simulink model "syt_a23"  (Simulink 7.0)
settings: Solver=ode3  StartTime=0.0  StopTime=10.0  FixedStep=0.01  RelTol=1e-3
settings Model: Creator=LAT04  LastModifiedBy=LAT04

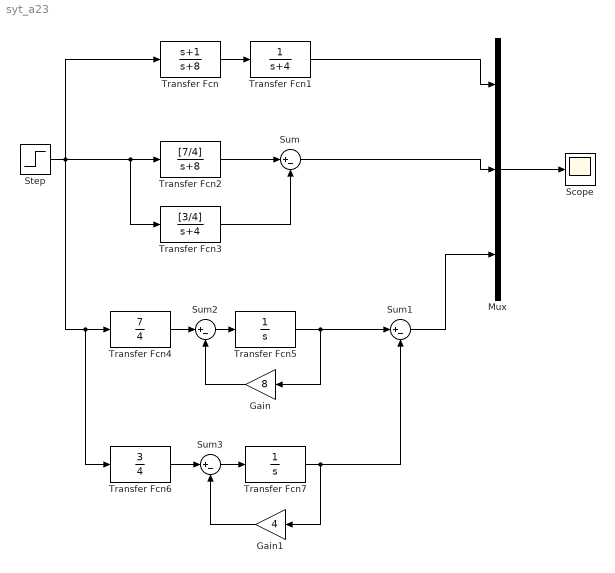
== system syt_a23 ==
  Gain : Gain  Orientation=left  Gain=8  ParameterDataType=sfix(16)  ParameterScaling=2^0  OutDataType=sfix(16)  OutScaling=2^0
  Gain1 : Gain  Orientation=left  Gain=4  ParameterDataType=sfix(16)  ParameterScaling=2^0  OutDataType=sfix(16)  OutScaling=2^0
  Mux : Mux  Inputs=3
  Scope : Scope
  Step : Step  SampleTime=0
  Sum{,1..3} (4 alike) : Sum  Inputs=|+-  OutDataType=sfix(16)  OutScaling=2^0
  Transfer Fcn : TransferFcn  Numerator=[1 1]  Denominator=[1 8]
  Transfer Fcn1 : TransferFcn  Denominator=[1 4]
  Transfer Fcn2 : TransferFcn  Numerator=[7/4]  Denominator=[1 8]
  Transfer Fcn3 : TransferFcn  Numerator=[3/4]  Denominator=[1 4]
  Transfer Fcn4 : TransferFcn  Numerator=[7]  Denominator=[4]
  Transfer Fcn5 : TransferFcn  Denominator=[1 0]
  Transfer Fcn6 : TransferFcn  Numerator=[3]  Denominator=[4]
  Transfer Fcn7 : TransferFcn  Denominator=[1 0]
  wires:
  Step/1 -> Transfer Fcn/1, Transfer Fcn2/1, Transfer Fcn3/1, Transfer Fcn4/1, Transfer Fcn6/1
  Transfer Fcn/1 -> Transfer Fcn1/1
  Transfer Fcn1/1 -> Mux/1
  Transfer Fcn2/1 -> Sum/1
  Transfer Fcn3/1 -> Sum/2
  Sum2/1 -> Transfer Fcn5/1
  Transfer Fcn4/1 -> Sum2/1
  Transfer Fcn5/1 -> Gain/1, Sum1/1
  Gain/1 -> Sum2/2
  Transfer Fcn6/1 -> Sum3/1
  Sum3/1 -> Transfer Fcn7/1
  Gain1/1 -> Sum3/2
  Transfer Fcn7/1 -> Gain1/1, Sum1/2
  Mux/1 -> Scope/1
  Sum/1 -> Mux/2
  Sum1/1 -> Mux/3
